simulink model "UPI_CC_3ph_4w_seq_23b"  (R2023b)
settings: Solver=FixedStepDiscrete  StartTime=0.0  StopTime=15  FixedStep=Ts_Power  MaxStep=1e-4  RelTol=1e-3
InitFcn:
  | run PI_OL_vs_UPI_CC_sec_ini;
undefined symbols (not defined in the file): C_2, DiscIntNeverNeededParam, K_i_pll, K_iv, K_p_pll, Ki_i, Kp_i, Kp_v, L_n, L_s2, L_t, L_t2, params_cc, params_pi_cc, params_pi_vc, params_vc_cc, R_d2, R_n, R_s2, R_t2, S_b, Ts_Control, Ts_Power, v_dc
libraries: spsFirstOrderFilterLib x7, spsThreePhaseSeriesRLCBranchLib x5, spsSeriesRLCLoadLib x5, spsUniversalBridgeLib x5, spsControlledVoltageSourceLib x3, spsThreePhaseVIMeasurementLib x3, eeGeneralControl x2, spsPower3phInstantaneousLib x2, spsSeriesRLCBranchLib x2, spsThreePhaseBreakerLib x2, spsRMSLib x1, simulink x1
(part 2 of 2)

== matlab function UPI_CC_3ph_4w_seq_23b/Control PI_VC/Voltage Control ==
  data: v_cdq_ref input; i_sdq input; i_tdq_ref output size=2; v_cdq input; omega input; params input; x input; dx output
function [i_tdq_ref,dx] = ctrl_vsc(v_cdq_ref,i_sdq,v_cdq,omega,params,x)

% parameters
C = params(7);
K_pv = params(8);
K_iv = params(9);

%References
v_cd_ref = v_cdq_ref(1);
v_cq_ref = v_cdq_ref(2);

i_sd = i_sdq(1);
i_sq = i_sdq(2);
v_cd = v_cdq(1);
v_cq = v_cdq(2);

% from the integrator to the states
xi_vcd = x(1);
xi_vcq = x(2);


% auxiliar
e_vcd = v_cd_ref - v_cd;
e_vcq = v_cq_ref - v_cq;

% derivatives
dxi_vcd = e_vcd;
dxi_vcq = e_vcq;


% auxiliar
u_d = K_pv*e_vcd + K_iv*xi_vcd;
u_q = K_pv*e_vcq + K_iv*xi_vcq;

% outputs
i_td_ref = (u_d - C*omega*v_cq + i_sd);
i_tq_ref = (u_q + C*omega*v_cd + i_sq);
i_tdq_ref = [i_td_ref ; i_tq_ref];


% from derivatives to the integrator
dx = [dxi_vcd;dxi_vcq];

== matlab function UPI_CC_3ph_4w_seq_23b/Control PI_CC/MATLAB Function4 ==
  data: theta input size=1; dq output; abc input
function dq  = fcn(theta,abc)
%#codegen

T_p = 2.0/3.0*[[ cos(theta), cos(theta-2.0/3.0*pi), cos(theta+2.0/3.0*pi)];
               [-sin(theta),-sin(theta-2.0/3.0*pi),-sin(theta+2.0/3.0*pi)]];
           
dq=T_p*abc;

== matlab function UPI_CC_3ph_4w_seq_23b/Control PI_CC/MATLAB Function5 ==
  data: theta input size=1; abc output size=3; dq input
function abc  = fcn(theta,dq)
%#codegen

T_p_inv = [[            cos(theta),            -sin(theta)];
           [ cos(theta-2.0/3.0*pi), -sin(theta-2.0/3.0*pi)];
           [ cos(theta+2.0/3.0*pi), -sin(theta+2.0/3.0*pi)]];
           
abc=T_p_inv*dq;

== matlab function UPI_CC_3ph_4w_seq_23b/Control PI_CC/PLL/MATLAB Function1 ==
  data: theta input size=1; dq output; abc input
function dq  = fcn(theta,abc)
%#codegen

T_p = 2.0/3.0*[[ cos(theta), cos(theta-2.0/3.0*pi), cos(theta+2.0/3.0*pi)];
               [-sin(theta),-sin(theta-2.0/3.0*pi),-sin(theta+2.0/3.0*pi)]];
           
dq=T_p*abc;

== matlab function UPI_CC_3ph_4w_seq_23b/Control PI_CC/VSG ==
  data: p_m_ref input; q_s_ref input; i_sdq input; i_sdq_ref output size=2; omega_rads output; v_sdq input; params input; omega_base input; x input; dx output
function [i_sdq_ref,omega_rads,dx] = ctrl_3(p_m_ref,q_s_ref,i_sdq,v_sdq,params,omega_base,x)
%Initialization
i_sdq_ref = [0;0];
fault_flag = 0;
e_0 = 1.0;

% parameters
S_b = params(1);
U_b = params(2);
K_p = params(3);
T_p = params(4);
K_q = params(5);
T_q = params(6);
X = params(7);
R = params(8);

%Base value
I_b = S_b/(sqrt(3)*U_b);
I_bdq = I_b*sqrt(2); 
U_bdq = U_b*(sqrt(2/3));

%Current and voltage in pu
i_sd = i_sdq(1)/I_bdq; % input in SI that is coverted to pu
i_sq = i_sdq(2)/I_bdq; % input in SI that is coverted to pu
v_sd = v_sdq(1)/U_bdq; % input in SI that is coverted to pu
v_sq = v_sdq(2)/U_bdq; % input in SI that is coverted to pu

%Active power en pu
p_s = i_sd*v_sd + i_sq*v_sq; % pu
q_s = i_sd*v_sq - i_sq*v_sd; % pu 

% from the integrator to the states
phi  = x(1);
xi_p = x(2);
xi_q = x(3);
omega_fil = x(4);

%error of active and reactive power
epsilon_p = (p_m_ref - p_s)*(1.0-fault_flag);
epsilon_q = q_s_ref - q_s;

%omega VSG
omega = K_p*(epsilon_p + xi_p/T_p) + omega_base; 
omega_rads = 2.0*pi*50.0*omega;
%Derivative outputs
dphi =  omega_rads;
dxi_p = epsilon_p;
dxi_q = epsilon_q; 
domega_rads = 1.0/1.0*(2.0*pi*50.0*omega - omega_fil);

%Voltage increase
DV =   K_q*(epsilon_q + xi_q/T_q); 

%Saturation of DV
DV_sat = DV;
if DV_sat > 0.1 
    DV_sat = 0.1;
    dxi_q = 0.0;
end
if DV_sat < -0.1 
    DV_sat = -0.1;
    dxi_q = 0.0;
end   

%Electromotive force of VSG
e = e_0 + DV_sat; 

%Virtual impdance
i_sd = -(X*e + R*v_sd + X*v_sq)/(R^2 + X^2);
i_sq = -(R*e + R*v_sq - X*v_sd)/(R^2 + X^2);

%Current references in A
i_sdq_ref(1) = i_sd*I_bdq;
i_sdq_ref(2) = i_sq*I_bdq;


% from derivatives to the integrator
dx = [dphi;dxi_p;dxi_q;domega_rads];

== matlab function UPI_CC_3ph_4w_seq_23b/Seq_Decom /MATLAB Function ==
  data: alpha input; albe_pos output size=2; beta input; albe_neg output size=2
function [albe_pos,albe_neg] = fcn(alpha,beta)

alpha_pos = 0.5*(alpha(1) - beta(2));
beta_pos = 0.5*(beta(1) + alpha(2));

alpha_neg = 0.5*(alpha(1) + beta(2));
beta_neg = 0.5*(beta(1) - alpha(2));

albe_pos = [alpha_pos;beta_pos];
albe_neg = [alpha_neg;beta_neg];

== matlab function UPI_CC_3ph_4w_seq_23b/MATLAB Function1 ==
  data: theta input size=1; abc output size=3; dq input
function abc  = fcn(theta,dq)
%#codegen

T_p_inv = [[            cos(theta),            -sin(theta)];
           [ cos(theta-2.0/3.0*pi), -sin(theta-2.0/3.0*pi)];
           [ cos(theta+2.0/3.0*pi), -sin(theta+2.0/3.0*pi)]];
           
abc=T_p_inv*dq;

== matlab function UPI_CC_3ph_4w_seq_23b/MATLAB Function2 ==
  data: theta input size=1; abc output size=3; dq input
function abc  = fcn(theta,dq)
%#codegen

T_p_inv = [[            cos(theta),            -sin(theta)];
           [ cos(theta-2.0/3.0*pi), -sin(theta-2.0/3.0*pi)];
           [ cos(theta+2.0/3.0*pi), -sin(theta+2.0/3.0*pi)]];
           
abc=T_p_inv*dq;

== matlab function UPI_CC_3ph_4w_seq_23b/Seq_Decom /MATLAB Function3 ==
  data: theta input size=1; dq output; abc input
function dq  = fcn(theta,abc)
%#codegen

T_p = 2.0/3.0*[[ cos(theta), cos(theta-2.0/3.0*pi), cos(theta+2.0/3.0*pi)];
               [-sin(theta),-sin(theta-2.0/3.0*pi),-sin(theta+2.0/3.0*pi)]];
           
dq=T_p*abc;

== matlab function UPI_CC_3ph_4w_seq_23b/Seq_Decom /alpha-beta_fasea_LPF1/MATLAB Function2 ==
  data: u1 input; u1_k_1 input; omega input; y1_k_1 input; y1_k output; y2_k_1 input; y2_k output
function [y1_k,y2_k]  = fcn(u1,u1_k_1,omega,y1_k_1,y2_k_1)


Ts_Control = 50e-6;
%y = x
%y1_k = (u1*omega + exp(-omega)*y1_k_1);
y1_k = ((u1 + u1_k_1)*omega*Ts_Control - (omega*Ts_Control-2)*y1_k_1)/(omega*Ts_Control + 2);

u2 = y1_k;
u2_k_1 = y1_k_1;

%y2_k = (u2*omega + exp(-omega)*y2_k_1);
y2_k = ((u2 + u2_k_1)*omega*Ts_Control - (omega*Ts_Control-2)*y2_k_1)/(omega*Ts_Control + 2);

== matlab function UPI_CC_3ph_4w_seq_23b/Seq_Decom 1/MATLAB Function ==
  data: alpha input; albe_pos output size=2; beta input; albe_neg output size=2
function [albe_pos,albe_neg] = fcn(alpha,beta)

alpha_pos = 0.5*(alpha(1) - beta(2));
beta_pos = 0.5*(beta(1) + alpha(2));

alpha_neg = 0.5*(alpha(1) + beta(2));
beta_neg = 0.5*(beta(1) - alpha(2));

albe_pos = [alpha_pos;beta_pos];
albe_neg = [alpha_neg;beta_neg];

== matlab function UPI_CC_3ph_4w_seq_23b/Seq_Decom 1/MATLAB Function3 ==
  data: theta input size=1; dq output; abc input
function dq  = fcn(theta,abc)
%#codegen

T_p = 2.0/3.0*[[ cos(theta), cos(theta-2.0/3.0*pi), cos(theta+2.0/3.0*pi)];
               [-sin(theta),-sin(theta-2.0/3.0*pi),-sin(theta+2.0/3.0*pi)]];
           
dq=T_p*abc;

== matlab function UPI_CC_3ph_4w_seq_23b/Control PI_VC/Current Control ==
  data: i_tdq_ref input; i_tdq input; eta_dq output size=2; v_cdq input; v_dc input; omega input; params input; x input; dx output
function [eta_dq,dx] = ctrl_vsc(i_tdq_ref,i_tdq,v_cdq,v_dc,omega,params,x)

% parameters
L_t = params(2);
K_pi = params(5);
K_ii = params(6);

%References
i_td_ref = i_tdq_ref(1);
i_tq_ref = i_tdq_ref(2);

i_td = i_tdq(1);
i_tq = i_tdq(2);
v_cd = v_cdq(1);
v_cq = v_cdq(2);

% from the integrator to the states
xi_itd = x(1);
xi_itq = x(2);


% auxiliar
e_itd = i_td_ref - i_td;
e_itq = i_tq_ref - i_tq;

% derivatives
dxi_itd = e_itd;
dxi_itq = e_itq;


% auxiliar
u_d = K_pi*e_itd + K_ii*xi_itd;
u_q = K_pi*e_itq + K_ii*xi_itq;
L = L_t;

% outputs
eta_d = 2/v_dc*(u_d - L*omega*i_tq + v_cd);
eta_q = 2/v_dc*(u_q + L*omega*i_td + v_cq);
eta_dq = [eta_d ; eta_q];


% from derivatives to the integrator
dx = [dxi_itd;dxi_itq];

== matlab function UPI_CC_3ph_4w_seq_23b/Control PI_CC/MATLAB Function1 ==
  data: theta input size=1; dq output; abc input
function dq  = fcn(theta,abc)
%#codegen

T_p = 2.0/3.0*[[ cos(theta), cos(theta-2.0/3.0*pi), cos(theta+2.0/3.0*pi)];
               [-sin(theta),-sin(theta-2.0/3.0*pi),-sin(theta+2.0/3.0*pi)]];
           
dq=T_p*abc;

== matlab function UPI_CC_3ph_4w_seq_23b/Seq_Decom 1/alpha-beta_fasea_LPF/MATLAB Function2 ==
  data: u1 input; u1_k_1 input; omega input; y1_k_1 input; y1_k output; y2_k_1 input; y2_k output
function [y1_k,y2_k]  = fcn(u1,u1_k_1,omega,y1_k_1,y2_k_1)


Ts_Control = 50e-6;
%y = x
%y1_k = (u1*omega + exp(-omega)*y1_k_1);
y1_k = ((u1 + u1_k_1)*omega*Ts_Control - (omega*Ts_Control-2)*y1_k_1)/(omega*Ts_Control + 2);

u2 = y1_k;
u2_k_1 = y1_k_1;

%y2_k = (u2*omega + exp(-omega)*y2_k_1);
y2_k = ((u2 + u2_k_1)*omega*Ts_Control - (omega*Ts_Control-2)*y2_k_1)/(omega*Ts_Control + 2);

== matlab function UPI_CC_3ph_4w_seq_23b/Seq_Decom 1/alpha-beta_fasea_LPF1/MATLAB Function2 ==
  data: u1 input; u1_k_1 input; omega input; y1_k_1 input; y1_k output; y2_k_1 input; y2_k output
function [y1_k,y2_k]  = fcn(u1,u1_k_1,omega,y1_k_1,y2_k_1)


Ts_Control = 50e-6;
%y = x
%y1_k = (u1*omega + exp(-omega)*y1_k_1);
y1_k = ((u1 + u1_k_1)*omega*Ts_Control - (omega*Ts_Control-2)*y1_k_1)/(omega*Ts_Control + 2);

u2 = y1_k;
u2_k_1 = y1_k_1;

%y2_k = (u2*omega + exp(-omega)*y2_k_1);
y2_k = ((u2 + u2_k_1)*omega*Ts_Control - (omega*Ts_Control-2)*y2_k_1)/(omega*Ts_Control + 2);

== matlab function UPI_CC_3ph_4w_seq_23b/albe-->dq/MATLAB Function1 ==
  data: theta input size=1; dq output; abc input
function dq  = fcn(theta,abc)
%#codegen

T_p = 2.0/3.0*[[ cos(theta), cos(theta-2.0/3.0*pi), cos(theta+2.0/3.0*pi)];
               [-sin(theta),-sin(theta-2.0/3.0*pi),-sin(theta+2.0/3.0*pi)]];
           
dq=T_p*abc;

== matlab function UPI_CC_3ph_4w_seq_23b/albe-->dq/MATLAB Function5 ==
  data: theta input size=1; abc output size=3; dq input
function abc  = fcn(theta,dq)
%#codegen

T_p_inv = [[            cos(theta),            -sin(theta)];
           [ cos(theta-2.0/3.0*pi), -sin(theta-2.0/3.0*pi)];
           [ cos(theta+2.0/3.0*pi), -sin(theta+2.0/3.0*pi)]];
           
abc=T_p_inv*dq;

== matlab function UPI_CC_3ph_4w_seq_23b/Seq_Decom /alpha-beta_fasea_LPF/MATLAB Function2 ==
  data: u1 input; u1_k_1 input; omega input; y1_k_1 input; y1_k output; y2_k_1 input; y2_k output
function [y1_k,y2_k]  = fcn(u1,u1_k_1,omega,y1_k_1,y2_k_1)


Ts_Control = 50e-6;
%y = x
%y1_k = (u1*omega + exp(-omega)*y1_k_1);
y1_k = ((u1 + u1_k_1)*omega*Ts_Control - (omega*Ts_Control-2)*y1_k_1)/(omega*Ts_Control + 2);

u2 = y1_k;
u2_k_1 = y1_k_1;

%y2_k = (u2*omega + exp(-omega)*y2_k_1);
y2_k = ((u2 + u2_k_1)*omega*Ts_Control - (omega*Ts_Control-2)*y2_k_1)/(omega*Ts_Control + 2);

== matlab function UPI_CC_3ph_4w_seq_23b/Control PI_CC/MATLAB Function ==
  data: i_s_abc input; i_s_abc_ref output; time input
function i_s_abc_ref = fcn(i_s_abc,time)
i_s_abc_ref = [0;0];

if time >1
    i_s_abc_ref = [i_s_abc(1);i_s_abc(2)];
end

== matlab function UPI_CC_3ph_4w_seq_23b/Control PI_VC/PLL/MATLAB Function1 ==
  data: theta input size=1; dq output; abc input
function dq  = fcn(theta,abc)
%#codegen

T_p = 2.0/3.0*[[ cos(theta), cos(theta-2.0/3.0*pi), cos(theta+2.0/3.0*pi)];
               [-sin(theta),-sin(theta-2.0/3.0*pi),-sin(theta+2.0/3.0*pi)]];
           
dq=T_p*abc;

== matlab function UPI_CC_3ph_4w_seq_23b/Control PI_VC/VSG ==
  data: e_0 input; p_m_ref input; q_s_ref input; i_sdq input; v_sdq input; v_mdq_ref output size=2; omega_rads output; params input; omega_base input; x input; dx output
function [v_mdq_ref,omega_rads,dx] = ctrl_3(e_0,p_m_ref,q_s_ref,i_sdq,v_sdq,params,omega_base,x)
%Initialization
v_mdq_ref = [0;0];
fault_flag = 0;

% parameters
S_b = params(1);
U_b = params(2);
K_p = params(3);
T_p = params(4);
K_q = params(5);
T_q = params(6);
X = params(7);
R = params(8);

%Base value
I_b = S_b/(sqrt(3)*U_b);
I_bdq = I_b*sqrt(2); 
U_bdq = U_b*(sqrt(2/3));

%Current and voltage in pu

v_sd = v_sdq(1)/U_bdq; % input in SI that is coverted to pu
v_sq = v_sdq(2)/U_bdq; % input in SI that is coverted to pu
i_sd = i_sdq(1)/I_bdq; % input in SI that is coverted to pu
i_sq = i_sdq(2)/I_bdq; % input in SI that is coverted to pu
%Active power en pu
p_s = i_sd*v_sd + i_sq*v_sq; % pu
q_s = i_sd*v_sq - i_sq*v_sd; % pu 

% from the integrator to the states
phi  = x(1);
xi_p = x(2);
xi_q = x(3);
omega_fil = x(4);

%error of active and reactive power
epsilon_p = (p_m_ref - p_s)*(1.0-fault_flag);
epsilon_q = q_s_ref - q_s;

%omega VSG
omega = K_p*(epsilon_p + xi_p/T_p) + omega_base; 
omega_rads = 2.0*pi*50.0*omega;
%Derivative outputs
dphi =  omega_rads;
dxi_p = epsilon_p;
dxi_q = epsilon_q; 
domega_rads = 1.0/1.0*(2.0*pi*50.0*omega - omega_fil);

%Voltage increase
DV =   K_q*(epsilon_q + xi_q/T_q*1); 

%Saturation of DV
DV_sat = DV;
if DV_sat > 0.1 
    DV_sat = 0.1;
    dxi_q = 0.0;
end
if DV_sat < -0.1 
    DV_sat = -0.1;
    dxi_q = 0.0;
end   

%Electromotive force of VSG
e = e_0 + DV_sat; 
e_d =0;
e_q = -e;
%Virtual impdance
v_md = e_d - (R*i_sd - X*i_sq) ;
v_mq = e_q - (X*i_sd + R*i_sq) ;

%Current references in A
v_mdq_ref(1) = v_md*U_bdq;
v_mdq_ref(2) = v_mq*U_bdq;


% from derivatives to the integrator
dx = [dphi;dxi_p;dxi_q;domega_rads];

== matlab function UPI_CC_3ph_4w_seq_23b/Control PI_VC/MATLAB Function3 ==
  data: theta input size=1; dq output; abc input
function dq  = fcn(theta,abc)
%#codegen

T_p = 2.0/3.0*[[ cos(theta), cos(theta-2.0/3.0*pi), cos(theta+2.0/3.0*pi)];
               [-sin(theta),-sin(theta-2.0/3.0*pi),-sin(theta+2.0/3.0*pi)]];
           
dq=T_p*abc;

== matlab function UPI_CC_3ph_4w_seq_23b/Control PI_VC/MATLAB Function4 ==
  data: theta input size=1; dq output; abc input
function dq  = fcn(theta,abc)
%#codegen

T_p = 2.0/3.0*[[ cos(theta), cos(theta-2.0/3.0*pi), cos(theta+2.0/3.0*pi)];
               [-sin(theta),-sin(theta-2.0/3.0*pi),-sin(theta+2.0/3.0*pi)]];
           
dq=T_p*abc;

== matlab function UPI_CC_3ph_4w_seq_23b/Control PI_VC/MATLAB Function5 ==
  data: theta input size=1; abc output size=3; dq input
function abc  = fcn(theta,dq)
%#codegen

T_p_inv = [[            cos(theta),            -sin(theta)];
           [ cos(theta-2.0/3.0*pi), -sin(theta-2.0/3.0*pi)];
           [ cos(theta+2.0/3.0*pi), -sin(theta+2.0/3.0*pi)]];
           
abc=T_p_inv*dq;

== matlab function UPI_CC_3ph_4w_seq_23b/Control PI_CC/Current Control ==
  data: i_sdq_ref input; i_sdq input; eta_dq output size=2; v_sdq input; v_dc input; omega input; params input; x input; dx output
function [eta_dq,dx] = ctrl_vsc(i_sdq_ref,i_sdq,v_sdq,v_dc,omega,params,x)

% parameters
L_t = params(2);
L_s = params(4);
K_p = params(5);
K_i = params(6);

%References
i_sd_ref = i_sdq_ref(1);
i_sq_ref = i_sdq_ref(2);

i_sd = i_sdq(1);
i_sq = i_sdq(2);
v_sd = v_sdq(1);
v_sq = v_sdq(2);

% from the integrator to the states
xi_isd = x(1);
xi_isq = x(2);


% auxiliar
e_isd = i_sd_ref - i_sd;
e_isq = i_sq_ref - i_sq;

% derivatives
dxi_isd = e_isd;
dxi_isq = e_isq;


% auxiliar
u_d = K_p*e_isd + K_i*xi_isd;
u_q = K_p*e_isq + K_i*xi_isq;
L = L_t + L_s ;

% outputs
eta_d = 2/v_dc*(u_d +  - L*omega*i_sq + v_sd);
eta_q = 2/v_dc*(u_q +  + L*omega*i_sd + v_sq);
eta_dq = [eta_d ; eta_q];


% from derivatives to the integrator
dx = [dxi_isd;dxi_isq];

== matlab function UPI_CC_3ph_4w_seq_23b/Control PI_CC/MATLAB Function3 ==
  data: theta input size=1; dq output; abc input
function dq  = fcn(theta,abc)
%#codegen

T_p = 2.0/3.0*[[ cos(theta), cos(theta-2.0/3.0*pi), cos(theta+2.0/3.0*pi)];
               [-sin(theta),-sin(theta-2.0/3.0*pi),-sin(theta+2.0/3.0*pi)]];
           
dq=T_p*abc;
